simulink subsystem "rss_DycCalc"  (R2023a)
settings: Solver=VariableStepAuto  StartTime=0.0  StopTime=inf  RelTol=1e-3
undefined symbols (not defined in the file): Genm_modePWMMode_C
libraries: lib_duty_cycle_waveform_generator x5
settings Model: DefaultTestHarness=rss_DutyCycleWaveformGenerator_thu  Creator=CAV2OFO  LastModifiedBy=xiaoqiang.yuan
settings OptimizationCC: ReuseModelBlockBuffer=off

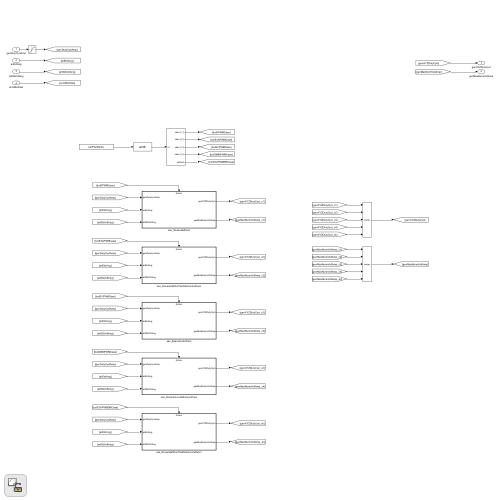
[thumbnail: Simulink's stored preview of the top-level diagram]
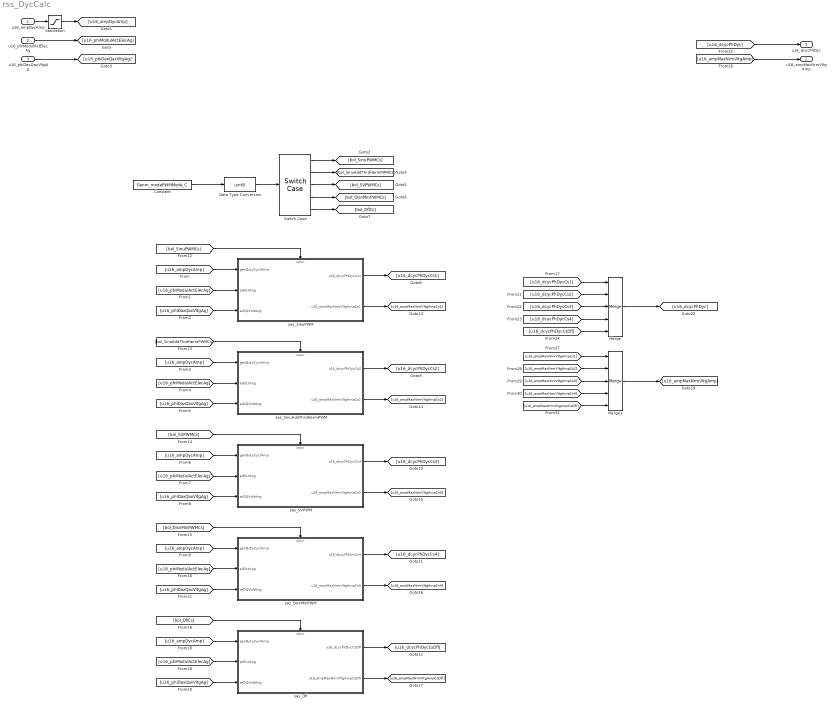
== system rss_DycCalc ==
  u16_ampDycAmp : Inport  OutDataTypeStr=dt_DutyCycl_u16p15b0
  u16_phiModulActElecAg : Inport  Port=2  OutDataTypeStr=dt_RadAng_u16r15b0
  u16_phiDaxQaxVltgAg : Inport  Port=3  OutDataTypeStr=dt_RadAng_u16r15b0
  Constant : Constant  Value=Genm_modePWMMode_C
  Data Type Conversion : DataTypeConversion  OutDataTypeStr=uint8  SaturateOnIntegerOverflow=off  RndMeth=Floor
  Merge : Merge  Inputs=5
  Merge1 : Merge  Inputs=5
  Saturation : Saturate  UpperLimit=1  LowerLimit=0
  Switch Case : SwitchCase  CaseConditions={1,2,3,4}
  sas_Dfl : Subsystem  TreatAsAtomicUnit=on
  sas_DisnMinPWM : Subsystem  TreatAsAtomicUnit=on
  sas_SVPWM : Subsystem  TreatAsAtomicUnit=on
  sas_SinuAddThrdHarmPWM : Subsystem  TreatAsAtomicUnit=on
  sas_SinuPWM : Subsystem  TreatAsAtomicUnit=on
  u16_dcycPhDyc : Outport  OutDataTypeStr=dt_DutyCycl_u16p15b0
  u16_ampMaxNrmVltgAmp : Outport  Port=2  OutDataTypeStr=dt_DutyCycl_u16p15b0
  wires:
  Merge1/1 -> [u16_ampMaxNrmVltgAmp]
  [u16_ampMaxNrmVltgAmpCsDfl] -> Merge1/5
  [u16_ampMaxNrmVltgAmpCs4] -> Merge1/4
  [u16_ampMaxNrmVltgAmpCs3] -> Merge1/3
  [u16_ampMaxNrmVltgAmpCs2] -> Merge1/2
  [u16_ampMaxNrmVltgAmpCs1] -> Merge1/1
  Merge/1 -> [u16_dcycPhDyc]
  [u16_dcycPhDycCsDfl] -> Merge/5
  [u16_dcycPhDycCs4] -> Merge/4
  [u16_dcycPhDycCs3] -> Merge/3
  [u16_dcycPhDycCs2] -> Merge/2
  [u16_dcycPhDycCs1] -> Merge/1
  sas_Dfl/2(u16_ampMaxNrmVltgAmpCsDfl) -> [u16_ampMaxNrmVltgAmpCsDfl]
  [u16_phiDaxQaxVltgAg] -> sas_Dfl/3(arDQVoltAng)
  sas_DisnMinPWM/2(u16_ampMaxNrmVltgAmpCs4) -> [u16_ampMaxNrmVltgAmpCs4]
  sas_SVPWM/2(u16_ampMaxNrmVltgAmpCs3) -> [u16_ampMaxNrmVltgAmpCs3]
  sas_SinuAddThrdHarmPWM/2(u16_ampMaxNrmVltgAmpCs2) -> [u16_ampMaxNrmVltgAmpCs2]
  sas_Dfl/1(u16_dcycPhDycCsDfl) -> [u16_dcycPhDycCsDfl]
  sas_DisnMinPWM/1(u16_dcycPhDycCs4) -> [u16_dcycPhDycCs4]
  sas_SVPWM/1(u16_dcycPhDycCs3) -> [u16_dcycPhDycCs3]
  sas_SinuAddThrdHarmPWM/1(u16_dcycPhDycCs2) -> [u16_dcycPhDycCs2]
  sas_SinuPWM/2(u16_ampMaxNrmVltgAmpCs1) -> [u16_ampMaxNrmVltgAmpCs1]
  sas_SinuPWM/1(u16_dcycPhDycCs1) -> [u16_dcycPhDycCs1]
  [u16_ampDycAmp] -> sas_Dfl/1(genDutyCyclAmp)
  [bol_DflCs] -> sas_Dfl/Action
  [u16_phiModulActElecAg] -> sas_Dfl/2(arElctAng)
  Switch Case/5 -> [bol_DflCs]
  Switch Case/4 -> [bol_DisnMinPWMCs]
  [bol_DisnMinPWMCs] -> sas_DisnMinPWM/Action
  [bol_SVPWMCs] -> sas_SVPWM/Action
  [bol_SinuAddThrdHarmPWMCs] -> sas_SinuAddThrdHarmPWM/Action
  [bol_SinuPWMCs] -> sas_SinuPWM/Action
  Switch Case/3 -> [bol_SVPWMCs]
  Switch Case/2 -> [bol_SinuAddThrdHarmPWMCs]
  Switch Case/1 -> [bol_SinuPWMCs]
  [u16_ampDycAmp] -> sas_DisnMinPWM/1(genDutyCyclAmp)
  [u16_phiModulActElecAg] -> sas_DisnMinPWM/2(arElctAng)
  [u16_phiDaxQaxVltgAg] -> sas_DisnMinPWM/3(arDQVoltAng)
  [u16_ampDycAmp] -> sas_SVPWM/1(genDutyCyclAmp)
  [u16_phiModulActElecAg] -> sas_SVPWM/2(arElctAng)
  [u16_phiDaxQaxVltgAg] -> sas_SVPWM/3(arDQVoltAng)
  [u16_ampDycAmp] -> sas_SinuAddThrdHarmPWM/1(genDutyCyclAmp)
  [u16_phiModulActElecAg] -> sas_SinuAddThrdHarmPWM/2(arElctAng)
  [u16_phiDaxQaxVltgAg] -> sas_SinuAddThrdHarmPWM/3(arDQVoltAng)
  [u16_phiDaxQaxVltgAg] -> sas_SinuPWM/3(arDQVoltAng)
  [u16_phiModulActElecAg] -> sas_SinuPWM/2(arElctAng)
  [u16_ampDycAmp] -> sas_SinuPWM/1(genDutyCyclAmp)
  u16_phiDaxQaxVltgAg/1 -> [u16_phiDaxQaxVltgAg]
  u16_phiModulActElecAg/1 -> [u16_phiModulActElecAg]
  u16_ampDycAmp/1 -> Saturation/1
  Constant/1 -> Data Type Conversion/1
  [u16_ampMaxNrmVltgAmp] -> u16_ampMaxNrmVltgAmp/1
  [u16_dcycPhDyc] -> u16_dcycPhDyc/1
  Data Type Conversion/1 -> Switch Case/1
  Saturation/1 -> [u16_ampDycAmp]

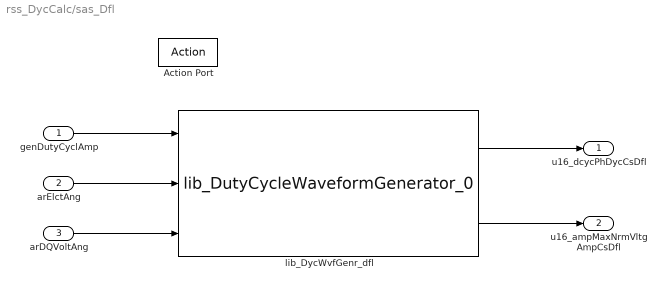
== system rss_DycCalc/sas_Dfl ==
  genDutyCyclAmp : Inport
  arElctAng : Inport  Port=2
  arDQVoltAng : Inport  Port=3
  Action Port : ActionPort
  lib_DycWvfGenr_dfl : lib_duty_cycle_waveform_generator/lib_DutyCycleWaveformGenerator_0  lb_parLktSize=1024  lb_parOmodFact=Gu16_facOvrModulFac_C  lb_parPWMMode=Sinusoidal plus third harmonics modulation
  u16_dcycPhDycCsDfl : Outport
  u16_ampMaxNrmVltgAmpCsDfl : Outport  Port=2
  wires:
  lib_DycWvfGenr_dfl/2 -> u16_ampMaxNrmVltgAmpCsDfl/1
  lib_DycWvfGenr_dfl/1 -> u16_dcycPhDycCsDfl/1
  arElctAng/1 -> lib_DycWvfGenr_dfl/2
  arDQVoltAng/1 -> lib_DycWvfGenr_dfl/3
  genDutyCyclAmp/1 -> lib_DycWvfGenr_dfl/1

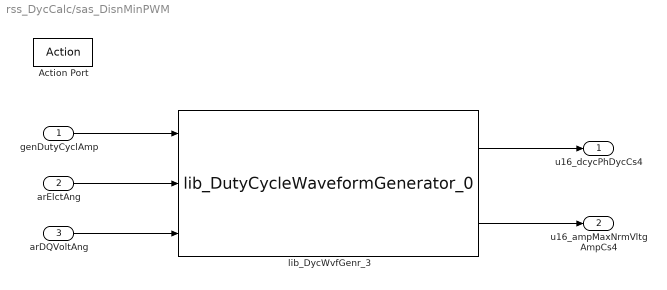
== system rss_DycCalc/sas_DisnMinPWM ==
  genDutyCyclAmp : Inport
  arElctAng : Inport  Port=2
  arDQVoltAng : Inport  Port=3
  Action Port : ActionPort
  lib_DycWvfGenr_3 : lib_duty_cycle_waveform_generator/lib_DutyCycleWaveformGenerator_0  lb_parLktSize=1024  lb_parOmodFact=Gu16_facOvrModulFac_C  lb_parPWMMode=Discontinuous minimum modulation
  u16_dcycPhDycCs4 : Outport
  u16_ampMaxNrmVltgAmpCs4 : Outport  Port=2
  wires:
  lib_DycWvfGenr_3/2 -> u16_ampMaxNrmVltgAmpCs4/1
  lib_DycWvfGenr_3/1 -> u16_dcycPhDycCs4/1
  arElctAng/1 -> lib_DycWvfGenr_3/2
  arDQVoltAng/1 -> lib_DycWvfGenr_3/3
  genDutyCyclAmp/1 -> lib_DycWvfGenr_3/1

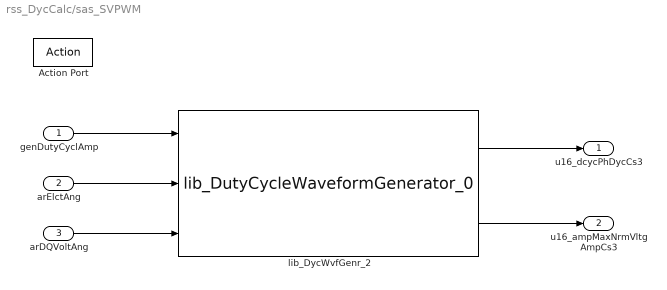
== system rss_DycCalc/sas_SVPWM ==
  genDutyCyclAmp : Inport
  arElctAng : Inport  Port=2
  arDQVoltAng : Inport  Port=3
  Action Port : ActionPort
  lib_DycWvfGenr_2 : lib_duty_cycle_waveform_generator/lib_DutyCycleWaveformGenerator_0  lb_parLktSize=1024  lb_parOmodFact=Gu16_facOvrModulFac_C  lb_parPWMMode=Space vector modulation
  u16_dcycPhDycCs3 : Outport
  u16_ampMaxNrmVltgAmpCs3 : Outport  Port=2
  wires:
  lib_DycWvfGenr_2/2 -> u16_ampMaxNrmVltgAmpCs3/1
  lib_DycWvfGenr_2/1 -> u16_dcycPhDycCs3/1
  arElctAng/1 -> lib_DycWvfGenr_2/2
  arDQVoltAng/1 -> lib_DycWvfGenr_2/3
  genDutyCyclAmp/1 -> lib_DycWvfGenr_2/1

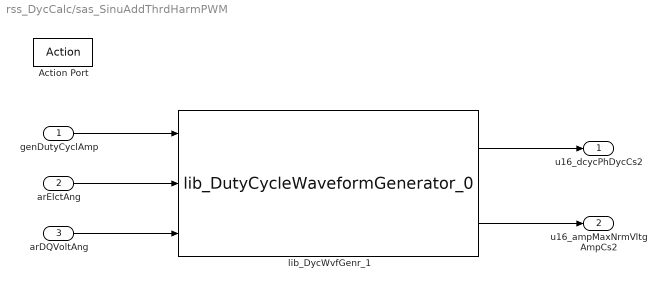
== system rss_DycCalc/sas_SinuAddThrdHarmPWM ==
  genDutyCyclAmp : Inport
  arElctAng : Inport  Port=2
  arDQVoltAng : Inport  Port=3
  Action Port : ActionPort
  lib_DycWvfGenr_1 : lib_duty_cycle_waveform_generator/lib_DutyCycleWaveformGenerator_0  lb_parLktSize=1024  lb_parOmodFact=Gu16_facOvrModulFac_C  lb_parPWMMode=Sinusoidal plus third harmonics modulation
  u16_dcycPhDycCs2 : Outport
  u16_ampMaxNrmVltgAmpCs2 : Outport  Port=2
  wires:
  lib_DycWvfGenr_1/2 -> u16_ampMaxNrmVltgAmpCs2/1
  lib_DycWvfGenr_1/1 -> u16_dcycPhDycCs2/1
  arElctAng/1 -> lib_DycWvfGenr_1/2
  arDQVoltAng/1 -> lib_DycWvfGenr_1/3
  genDutyCyclAmp/1 -> lib_DycWvfGenr_1/1

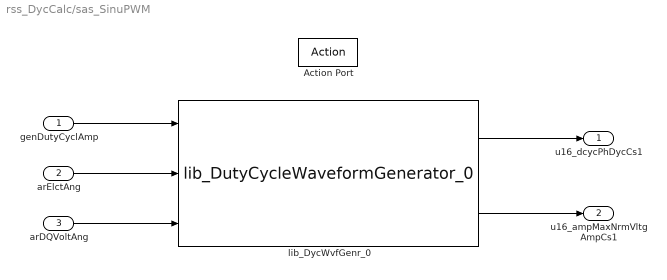
== system rss_DycCalc/sas_SinuPWM ==
  genDutyCyclAmp : Inport
  arElctAng : Inport  Port=2
  arDQVoltAng : Inport  Port=3
  Action Port : ActionPort
  lib_DycWvfGenr_0 : lib_duty_cycle_waveform_generator/lib_DutyCycleWaveformGenerator_0  lb_parLktSize=1024  lb_parOmodFact=Gu16_facOvrModulFac_C  lb_parPWMMode=Sinusoidal modulation
  u16_dcycPhDycCs1 : Outport
  u16_ampMaxNrmVltgAmpCs1 : Outport  Port=2
  wires:
  arDQVoltAng/1 -> lib_DycWvfGenr_0/3
  arElctAng/1 -> lib_DycWvfGenr_0/2
  genDutyCyclAmp/1 -> lib_DycWvfGenr_0/1
  lib_DycWvfGenr_0/2 -> u16_ampMaxNrmVltgAmpCs1/1
  lib_DycWvfGenr_0/1 -> u16_dcycPhDycCs1/1
